simulink model "vehicle_body_revised"  (R2020b)
settings: Solver=VariableStepAuto  StartTime=0.0  StopTime=10.0  RelTol=1e-3
libraries: sdl_lib x17, nesl_utility x8, autolibdatasheetbattery x1, autolibmappedmotor x1
settings Model: Creator=True  LastModifiedBy=True

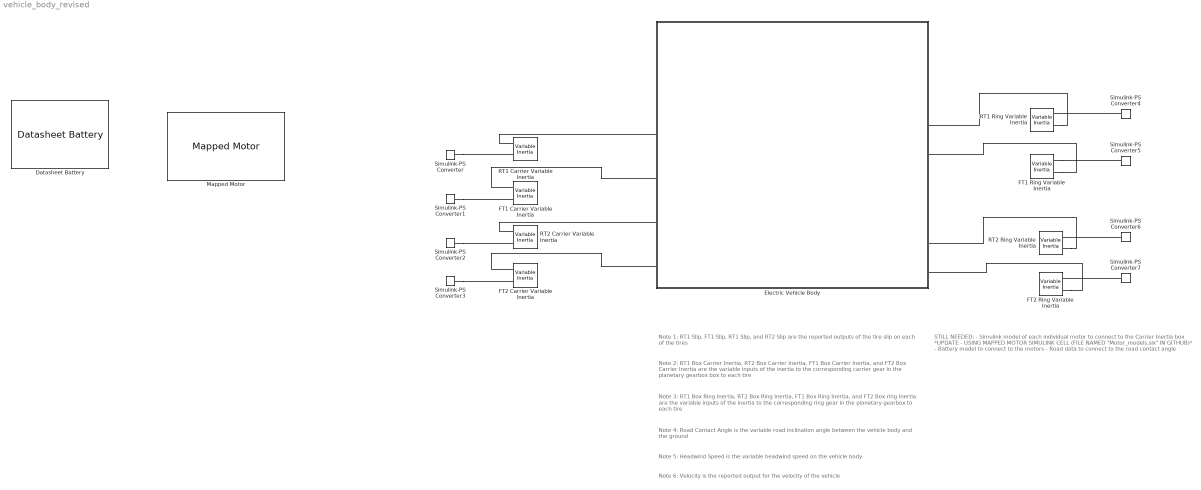
== system vehicle_body_revised ==
  note: STILL NEEDED:
      | - Simulink model of each individual motor to connect to the Carrier Inertia box *UPDATE - USING MAPPED MOTOR SIMULINK CELL (FILE NAMED "Motor_models.slx" IN GITHUB)*
      |
      | - Battery model to connect to the motors
      |
      | - Road data to connect to the road contact angle
  note: Note 6: Velocity is the reported output for the velocity of the vehicle
  note: Note 5: Headwind Speed is the variable headwind speed on the vehicle body
  note: Note 4: Road Contact Angle is the variable road inclination angle between the vehicle body and the ground
  note: Note 3: RT1 Box Ring Inertia, RT2 Box Ring Inertia, FT1 Box Ring Inertia, and FT2 Box ring Inertia are the variable inputs of the inertia to the corresponding ring gear in the planetary gearbox to each tire
  note: Note 2: RT1 Box Carrier Inertia, RT2 Box Carrier Inertia, FT1 Box Carrier Inertia, and FT2 Box Carrier Inertia are the variable inputs of the inertia to the corresponding carrier gear in the planetary gearbox box to each tire
  note: Note 1: RT1 Slip, FT1 Slip, RT1 Slip, and RT2 Slip are the reported outputs of the tire slip on each of the tires
  Datasheet Battery : autolibdatasheetbattery/Datasheet Battery  CapacityCtrl=Parameter  OutputVlt=Unfiltered  BattChargeMax=100  Em=[2.8 3.228 3.284 3.361 3.408 3.427 3.472 3.477 3.493 3.504 3.516 3.528 3.537 3.545 3.555 3.561 3.566 3.576 3.587 3.589 3.594 3.6 3.608 3.61 3.616 3.619 3.626 3.632 3.637 3.64 3.645 3.646 3.652 3.655 3.658 3.661 3.664 3.668 3.673 3.678 3.68 3.681 3.686 3.692 3.699 3.702 3.705 3.71 3.717 3.723 3.728 3.733 3.735 3.742 3.749 3.755 3.761 3.768 3.773 3.78 3.791 3.798 3.798 3.814 3.818 3.825 3.841 3.846 3.855 3.863 3.877 3.885 3.894 3.907 3.919 3.926 3.935 3.944 3.954 3.964 3.974 3.988 3.998 4.014 4.029 4.034 4.047 4.065 4.074 4.086 4.097 4.131 4.126 4.138 4.15 4.18 4.174 4.187 4.207 4.231 4.221]  CapLUTBp=[0 0.01 0.02 0.03 0.04 0.05 0.06 0.07 0.08 0.09 0.1 0.11 0.12 0.13 0.14 0.15 0.16 0.17 0.18 0.19 0.2 0.21 0.22 0.23 0.24 0.25 0.26 0.27 0.28 0.29 0.3 0.31 0.32 0.33 0.34 0.35 0.36 0.37 0.38 0.39 0.4 0.41 0.42 0.43 0.44 0.45 0.46 0.47 0.48 0.49 0.5 0.51 0.52 0.53 0.54 0.55 0.56 0.57 0.58 0.59 0.6 0.61 0.62 0.63 0.64 0.65 0.66 0.67 0.68 0.69 0.7 0.71 0.72 0.73 0.74 0.75 0.76 0.77 0.78 0.79 0.8 0.81 0.82 0.83 0.84 0.85 0.86 0.87 0.88 0.89 0.9 0.91 0.92 0.93 0.94 0.95 0.96 0.97 0.98 0.99 1]  RInt=[0.008846 0.009319 0.009027 0.00847 0.01032 0.01314;0.006389 0.006554 0.005553 0.005525 0.006043 0.007805;0.004364 0.004101 0.00406 0.003452 0.003846 0.004517;0.002031 0.002563 0.002532 0.00246 0.002716 0.003047;0.001443 0.001825 0.001795 0.001778 0.001924 0.002234;0.0005603 0.0007192 0.0006887 0.0007557 0.0007355 0.001014;0.001028 0.001338 0.001 0.001536 0.001546 0.002789]  BattTempBp=[243.1 253.1 263.1 273.1 283.1 298.1 313.1]  CapSOCBp=[0 0.2 0.4 0.6 0.8 1]  Ns=1  Np=1  BattCapInit=100  Tc=1/1000  Vinit=4.221  RefBlkName='autolibdatasheetbattery/Datasheet Battery'
      settings: SourceProductBaseCode=PW
  Electric Vehicle Body : Subsystem
  FT1 Carrier Variable Inertia : sdl_lib/Inertias & Loads/Variable Inertia  minimum_inertia=0.1 kg*m^2  L_specify=off  L_priority=High  L=0 m^2*kg/s  L_nominal_specify=off  L_nominal_unit=m^2*kg/s  L_nominal_value=1
      settings: SourceProductBaseCode=LD  InternalSimscapePortConfiguration="{\"Bottom\":[],\"Left\":[{\"id\":\"I\",\"label\":\"\",\"type\":\"input\"},{\"id\":\"A\",\"label\":\"\",\"type\":\"foundation.mechanical.rotational.rotational\"}],\"Right\":[],\"Top\":[]}"
  FT1 Ring Variable Inertia : sdl_lib/Inertias & Loads/Variable Inertia  minimum_inertia=0.1 kg*m^2  L_specify=off  L_priority=High  L=0 m^2*kg/s  L_nominal_specify=off  L_nominal_unit=m^2*kg/s  L_nominal_value=1
      settings: SourceProductBaseCode=LD  InternalSimscapePortConfiguration="{\"Bottom\":[],\"Left\":[{\"id\":\"I\",\"label\":\"\",\"type\":\"input\"},{\"id\":\"A\",\"label\":\"\",\"type\":\"foundation.mechanical.rotational.rotational\"}],\"Right\":[],\"Top\":[]}"
  FT2 Carrier Variable Inertia : sdl_lib/Inertias & Loads/Variable Inertia  minimum_inertia=0.1 kg*m^2  L_specify=off  L_priority=High  L=0 m^2*kg/s  L_nominal_specify=off  L_nominal_unit=m^2*kg/s  L_nominal_value=1
      settings: SourceProductBaseCode=LD  InternalSimscapePortConfiguration="{\"Bottom\":[],\"Left\":[{\"id\":\"I\",\"label\":\"\",\"type\":\"input\"},{\"id\":\"A\",\"label\":\"\",\"type\":\"foundation.mechanical.rotational.rotational\"}],\"Right\":[],\"Top\":[]}"
  FT2 Ring Variable Inertia : sdl_lib/Inertias & Loads/Variable Inertia  minimum_inertia=0.1 kg*m^2  L_specify=off  L_priority=High  L=0 m^2*kg/s  L_nominal_specify=off  L_nominal_unit=m^2*kg/s  L_nominal_value=1
      settings: SourceProductBaseCode=LD  InternalSimscapePortConfiguration="{\"Bottom\":[],\"Left\":[{\"id\":\"I\",\"label\":\"\",\"type\":\"input\"},{\"id\":\"A\",\"label\":\"\",\"type\":\"foundation.mechanical.rotational.rotational\"}],\"Right\":[],\"Top\":[]}"
  Mapped Motor : autolibmappedmotor/Mapped Motor  port_config=Torque  param_by=Tabulated torque-speed envelope  w_t=[ 0 375 750 800 ]  T_t=[0.09 0.08 0.07 0]  torque_max=.1  power_max=30  Tc=0.02  param_loss=Single efficiency measurement  eff=100  w_eff=375  T_eff=0.08  Piron=0  Pbase=0  w_eff_bp=[-8000 -4000 0 4000 8000]  T_eff_bp=[0 0.03 0.06 0.09]  Temp_eff_bp=[233.15 293.15 373.15]  losses_table=[1.49 1.67 2.21 3.10; 0.42 0.69 1.14 2.03; 0.06 0.24 0.78 1.68; 0.42 0.69 1.14 2.03; 1.49 1.67 2.21 3.10]  losses_table_3d=cat(3,[1.49 1.67 2.21 3.10; 0.42 0.69 1.14 2.03; 0.06 0.24 0.78 1.68; 0.42 0.69 1.14 2.03; 1.49 1.67 2.21 3.10],[1.49 1.67 2.21 3.10; 0.42 0.69 1.14 2.03; 0.06 0.24 0.78 1.68; 0.42 0.69 1.14 2.03; 1.49 1.67 2.21 3.10],[1.49 1.67 2.21 3.10; 0.42 0.69 1.14 2.03; 0.06 0.24 0.78 1.68; 0.42 0.69 1.14 2.03; 1.49 1.67 2.21 3.10])  efficiency_table=[95 95 95 95; 95 95 95 95; 95 95 95 95; 95 95 95 95; 95 95 95 95]  efficiency_table_3d=cat(3,[95 95 95 95; 95 95 95 95; 95 95 95 95; 95 95 95 95; 95 95 95 95],[95 95 95 95; 95 95 95 95; 95 95 95 95; 95 95 95 95; 95 95 95 95],[95 95 95 95; 95 95 95 95; 95 95 95 95; 95 95 95 95; 95 95 95 95])  J=5e-6  b=1e-5  omega_o=0  T_t_extended=[0 0.07 0.08 0.09 0.08 0.07 0]  w_t_extended=[-800 -750 -375 0 375 750 800]  KLossIron=0  KLossCopper=0  x_w_eff_vec=[-8000 -4000 0 4000 8000]  x_T_eff_vec=[-0.09 -0.06 -0.03 0 0.03 0.06 0.09]  x_tmp_eff_vec=[-0.09 -0.06 -0.03 0 0.03 0.06 0.09]  x_losses_mat=[3.1 2.21 1.67 1.49 1.67 2.21 3.1;2.03 1.14 0.69 0.42 0.69 1.14 2.03;1.68 0.78 0.24 0.06 0.24 0.78 1.68;2.03 1.14 0.69 0.42 0.69 1.14 2.03;3.1 2.21 1.67 1.49 1.67 2.21 3.1]  x_losses_mat_3d=[37.8947368421052 25.2631578947368 12.6315789473684 0 12 24 36;18.9473684210526 12.6315789473684 6.3157894736842 0 5.99999999999999 12 18;0 0 0 0 0 0 0;18 12 5.99999999999999 0 6.3157894736842 12.6315789473684 18.9473684210526;36 24 12 0 12.6315789473684 25.2631578947368 37.8947368421052]  CalLossMapData={}  CalLossWithTempMapData={}  aMode=1  RefBlkName='autolibmappedmotor/Mapped Motor'
      settings: SourceProductBaseCode=PW,MT,UV,VE,VP
  RT1 Carrier Variable Inertia : sdl_lib/Inertias & Loads/Variable Inertia  minimum_inertia=0.1 kg*m^2  L_specify=off  L_priority=High  L=0 m^2*kg/s  L_nominal_specify=off  L_nominal_unit=m^2*kg/s  L_nominal_value=1
      settings: SourceProductBaseCode=LD  InternalSimscapePortConfiguration="{\"Bottom\":[],\"Left\":[{\"id\":\"I\",\"label\":\"\",\"type\":\"input\"},{\"id\":\"A\",\"label\":\"\",\"type\":\"foundation.mechanical.rotational.rotational\"}],\"Right\":[],\"Top\":[]}"
  RT1 Ring Variable Inertia : sdl_lib/Inertias & Loads/Variable Inertia  minimum_inertia=0.1 kg*m^2  L_specify=off  L_priority=High  L=0 m^2*kg/s  L_nominal_specify=off  L_nominal_unit=m^2*kg/s  L_nominal_value=1
      settings: SourceProductBaseCode=LD  InternalSimscapePortConfiguration="{\"Bottom\":[],\"Left\":[{\"id\":\"I\",\"label\":\"\",\"type\":\"input\"},{\"id\":\"A\",\"label\":\"\",\"type\":\"foundation.mechanical.rotational.rotational\"}],\"Right\":[],\"Top\":[]}"
  RT2 Carrier Variable Inertia : sdl_lib/Inertias & Loads/Variable Inertia  minimum_inertia=0.1 kg*m^2  L_specify=off  L_priority=High  L=0 m^2*kg/s  L_nominal_specify=off  L_nominal_unit=m^2*kg/s  L_nominal_value=1
      settings: SourceProductBaseCode=LD  InternalSimscapePortConfiguration="{\"Bottom\":[],\"Left\":[{\"id\":\"I\",\"label\":\"\",\"type\":\"input\"},{\"id\":\"A\",\"label\":\"\",\"type\":\"foundation.mechanical.rotational.rotational\"}],\"Right\":[],\"Top\":[]}"
  RT2 Ring Variable Inertia : sdl_lib/Inertias & Loads/Variable Inertia  minimum_inertia=0.1 kg*m^2  L_specify=off  L_priority=High  L=0 m^2*kg/s  L_nominal_specify=off  L_nominal_unit=m^2*kg/s  L_nominal_value=1
      settings: SourceProductBaseCode=LD  InternalSimscapePortConfiguration="{\"Bottom\":[],\"Left\":[{\"id\":\"I\",\"label\":\"\",\"type\":\"input\"},{\"id\":\"A\",\"label\":\"\",\"type\":\"foundation.mechanical.rotational.rotational\"}],\"Right\":[],\"Top\":[]}"
  Simulink-PS Converter{,1..7} (8 alike) : nesl_utility/Simulink-PS Converter  PhysicalDomain=network_engine_domain  SubClassName=ps_input  LeftPortType=input  RightPortType=output  PseudoPeriodic=off  Frequencies=[]  NoiseDistribution=none  NoiseParameters=[]  Unit=1  AffineConversion=off  FilteringAndDerivatives=provide  SimscapeFilterOrder=1  InputFilterTimeConstant=0.001  UdotUserProvided=0
  connections:
  RT1 Carrier Variable Inertia/LConn2 -- Electric Vehicle Body/LConn3
  FT1 Carrier Variable Inertia/LConn2 -- Electric Vehicle Body/LConn4
  RT2 Carrier Variable Inertia/LConn2 -- Electric Vehicle Body/LConn5
  FT2 Carrier Variable Inertia/LConn2 -- Electric Vehicle Body/LConn6
  RT1 Ring Variable Inertia/LConn2 -- Electric Vehicle Body/RConn4
  FT1 Ring Variable Inertia/LConn2 -- Electric Vehicle Body/RConn5
  RT2 Ring Variable Inertia/LConn2 -- Electric Vehicle Body/RConn8
  FT2 Ring Variable Inertia/LConn2 -- Electric Vehicle Body/RConn9
  Simulink-PS Converter/RConn1 -- RT1 Carrier Variable Inertia/LConn1
  Simulink-PS Converter1/RConn1 -- FT1 Carrier Variable Inertia/LConn1
  Simulink-PS Converter2/RConn1 -- RT2 Carrier Variable Inertia/LConn1
  Simulink-PS Converter3/RConn1 -- FT2 Carrier Variable Inertia/LConn1
  Simulink-PS Converter4/RConn1 -- RT1 Ring Variable Inertia/LConn1
  FT1 Ring Variable Inertia/LConn1 -- Simulink-PS Converter5/RConn1
  Simulink-PS Converter6/RConn1 -- RT2 Ring Variable Inertia/LConn1
  Simulink-PS Converter7/RConn1 -- FT2 Ring Variable Inertia/LConn1

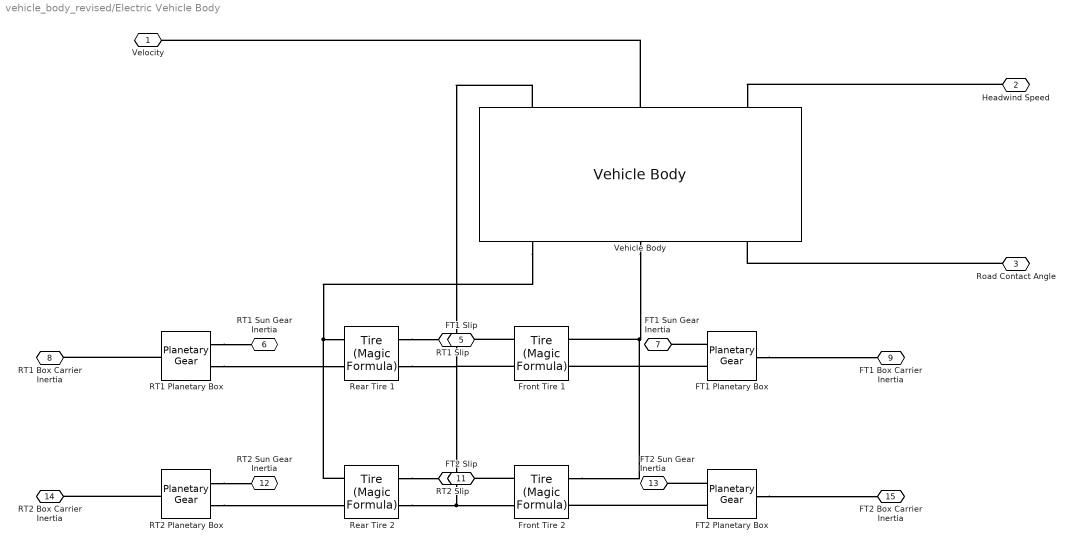
== system vehicle_body_revised/Electric Vehicle Body ==
  FT1 Planetary Box : sdl_lib/Gears/Planetary Gear  rs_ratio=2  friction_model=sdl.enum.gear_friction.none  mu_visc=[0, 0] N*m/(rad/s)  efficiency=[.96, .98]  temperature_TLU=[280, 300, 320] K  efficiency_sp_TLU=[.95, .9, .85]  efficiency_rp_TLU=[.95, .9, .85]  pwr_thr=[.001, .001] W  thermal_mass=50 J/K  T_init=300 K  model_inertia=simscape.enum.onoff.off  planet_inertia=0.001 kg*m^2
      settings: SourceProductBaseCode=LD
  FT2 Planetary Box : sdl_lib/Gears/Planetary Gear  rs_ratio=2  friction_model=sdl.enum.gear_friction.none  mu_visc=[0, 0] N*m/(rad/s)  efficiency=[.96, .98]  temperature_TLU=[280, 300, 320] K  efficiency_sp_TLU=[.95, .9, .85]  efficiency_rp_TLU=[.95, .9, .85]  pwr_thr=[.001, .001] W  thermal_mass=50 J/K  T_init=300 K  model_inertia=simscape.enum.onoff.off  planet_inertia=0.001 kg*m^2
      settings: SourceProductBaseCode=LD
  Front Tire 1 : sdl_lib/Tires & Vehicles/Tire (Magic Formula)  parameterization=sdl.enum.magic_tire_model.peak  F_z1=3000 N  F_x1=3500 N  kappa1=10  B_m=10  C_m=1.9  D_m=1  E_m=0.97  fz0=4000 N  p_Cx=1.685  p_Dx=[1.21, -.037]  p_Ex=[.344, .095, -.02, 0]  p_Kx=[21.51, -.163, .245]  p_Hx=[-.002, .002]  p_Vx=[0, 0]  v_tr_thr=0.1 m/s  r_e=0.3 m  model_compliance=0  stiffness=1e6 N/m  damping=1000 N/(m/s)  model_inertia=0  inertia=1 kg*m^2  initial_velocity=0 rad/s  model_resistance=0  resistance_model=1  coeff=0.015  p_tire=250e3 Pa  alpha=-0.003  beta=0.97  coeff_a=84e-4  coeff_b=6.2e-4 s/m  coeff_c=1.6e-4 s^2/m^2  v_thr=0.001 m/s
  Front Tire 2 : sdl_lib/Tires & Vehicles/Tire (Magic Formula)  parameterization=sdl.enum.magic_tire_model.peak  F_z1=3000 N  F_x1=3500 N  kappa1=10  B_m=10  C_m=1.9  D_m=1  E_m=0.97  fz0=4000 N  p_Cx=1.685  p_Dx=[1.21, -.037]  p_Ex=[.344, .095, -.02, 0]  p_Kx=[21.51, -.163, .245]  p_Hx=[-.002, .002]  p_Vx=[0, 0]  v_tr_thr=0.1 m/s  r_e=0.3 m  model_compliance=0  stiffness=1e6 N/m  damping=1000 N/(m/s)  model_inertia=0  inertia=1 kg*m^2  initial_velocity=0 rad/s  model_resistance=0  resistance_model=1  coeff=0.015  p_tire=250e3 Pa  alpha=-0.003  beta=0.97  coeff_a=84e-4  coeff_b=6.2e-4 s/m  coeff_c=1.6e-4 s^2/m^2  v_thr=0.001 m/s
  RT1 Planetary Box : sdl_lib/Gears/Planetary Gear  rs_ratio=2  friction_model=sdl.enum.gear_friction.none  mu_visc=[0, 0] N*m/(rad/s)  efficiency=[.96, .98]  temperature_TLU=[280, 300, 320] K  efficiency_sp_TLU=[.95, .9, .85]  efficiency_rp_TLU=[.95, .9, .85]  pwr_thr=[.001, .001] W  thermal_mass=50 J/K  T_init=300 K  model_inertia=simscape.enum.onoff.off  planet_inertia=0.001 kg*m^2
      settings: SourceProductBaseCode=LD
  RT2 Planetary Box : sdl_lib/Gears/Planetary Gear  rs_ratio=2  friction_model=sdl.enum.gear_friction.none  mu_visc=[0, 0] N*m/(rad/s)  efficiency=[.96, .98]  temperature_TLU=[280, 300, 320] K  efficiency_sp_TLU=[.95, .9, .85]  efficiency_rp_TLU=[.95, .9, .85]  pwr_thr=[.001, .001] W  thermal_mass=50 J/K  T_init=300 K  model_inertia=simscape.enum.onoff.off  planet_inertia=0.001 kg*m^2
      settings: SourceProductBaseCode=LD
  Rear Tire 1 : sdl_lib/Tires & Vehicles/Tire (Magic Formula)  parameterization=sdl.enum.magic_tire_model.peak  F_z1=3000 N  F_x1=3500 N  kappa1=10  B_m=10  C_m=1.9  D_m=1  E_m=0.97  fz0=4000 N  p_Cx=1.685  p_Dx=[1.21, -.037]  p_Ex=[.344, .095, -.02, 0]  p_Kx=[21.51, -.163, .245]  p_Hx=[-.002, .002]  p_Vx=[0, 0]  v_tr_thr=0.1 m/s  r_e=0.3 m  model_compliance=0  stiffness=1e6 N/m  damping=1000 N/(m/s)  model_inertia=0  inertia=1 kg*m^2  initial_velocity=0 rad/s  model_resistance=0  resistance_model=1  coeff=0.015  p_tire=250e3 Pa  alpha=-0.003  beta=0.97  coeff_a=84e-4  coeff_b=6.2e-4 s/m  coeff_c=1.6e-4 s^2/m^2  v_thr=0.001 m/s
  Rear Tire 2 : sdl_lib/Tires & Vehicles/Tire (Magic Formula)  parameterization=sdl.enum.magic_tire_model.peak  F_z1=3000 N  F_x1=3500 N  kappa1=10  B_m=10  C_m=1.9  D_m=1  E_m=0.97  fz0=4000 N  p_Cx=1.685  p_Dx=[1.21, -.037]  p_Ex=[.344, .095, -.02, 0]  p_Kx=[21.51, -.163, .245]  p_Hx=[-.002, .002]  p_Vx=[0, 0]  v_tr_thr=0.1 m/s  r_e=0.3 m  model_compliance=0  stiffness=1e6 N/m  damping=1000 N/(m/s)  model_inertia=0  inertia=1 kg*m^2  initial_velocity=0 rad/s  model_resistance=0  resistance_model=1  coeff=0.015  p_tire=250e3 Pa  alpha=-0.003  beta=0.97  coeff_a=84e-4  coeff_b=6.2e-4 s/m  coeff_c=1.6e-4 s^2/m^2  v_thr=0.001 m/s
  Vehicle Body : sdl_lib/Tires & Vehicles/Vehicle Body  mass=1200 kg  n_w=2  x_f=1.4 m  x_r=1.6 m  y_c=0.5 m  mass_var=simscape.enum.onoff.off  model_pitch=simscape.enum.onoff.off  inertia=4000 kg*m^2  suspension_model=sdl.enum.linearTLU.linear  k_f=1e4 N/m  b_f=1e4 N/(m/s)  k_r=1e4 N/m  b_r=1e4 N/(m/s)  k_f_TLU=[-2000, -1000, 0, 1000, 2000] N  x_f_TLU=[-.4, -.2, 0, .2, .4] m  b_f_TLU=[-200, -100, 0, 100, 200] N  v_f_TLU=[-4, -2, 0, 2, 4] m/s  k_r_TLU=[-2000, -1000, 0, 1000, 2000] N  x_r_TLU=[-.4, -.2, 0, .2, .4] m  b_r_TLU=[-200, -100, 0, 100, 200] N  v_r_TLU=[-4, -2, 0, 2, 4] m/s  interp_method=simscape.enum.interpolation.linear  extrap_method=simscape.enum.extrapolation.linear  model_hardstop=simscape.enum.onoff.off  upper_bound_f=.25 m  lower_bound_f=-.25 m  stop_k_f=1e6 N/m  stop_b_f=150 N/(m/s)  upper_bound_r=.25 m  lower_bound_r=-.25 m  stop_k_r=1e6 N/m  stop_b_r=150 N/(m/s)  initial_pitch=0 rad  initial_pitch_rate=0 rad/s  g=9.81 m/s^2  liftoff_warning=simscape.enum.onoff.off  area=3 m^2  Cd=0.4  rho=1.18 kg/m^3  v_specify=off  v_priority=High  v=0 m/s  v_nominal_specify=off  v_nominal_unit=m/s  v_nominal_value=1
  Velocity : PMIOPort  Side=Left
  Headwind Speed : PMIOPort  Port=2  Side=Left
  Road Contact Angle : PMIOPort  Port=3  Side=Right
  RT1 Slip : PMIOPort  Port=4  Side=Right
  FT1 Slip : PMIOPort  Port=5  Side=Right
  RT1 Sun Gear Inertia : PMIOPort  Port=6  Side=Right
  FT1 Sun Gear Inertia : PMIOPort  Port=7  Side=Right
  RT1 Box Carrier Inertia : PMIOPort  Port=8  Side=Left
  FT1 Box Carrier Inertia : PMIOPort  Port=9  Side=Left
  RT2 Slip : PMIOPort  Port=10  Side=Right
  FT2 Slip : PMIOPort  Port=11  Side=Right
  RT2 Sun Gear Inertia : PMIOPort  Port=12  Side=Right
  FT2 Sun Gear Inertia : PMIOPort  Port=13  Side=Right
  RT2 Box Carrier Inertia : PMIOPort  Port=14  Side=Left
  FT2 Box Carrier Inertia : PMIOPort  Port=15  Side=Left
  connections:
  Front Tire 2/LConn1 -- Front Tire 1/LConn1 -- Vehicle Body/RConn2
  Rear Tire 2/LConn1 -- Rear Tire 1/LConn1 -- Vehicle Body/RConn1
  Road Contact Angle/RConn1 -- Vehicle Body/RConn3
  FT2 Planetary Box/RConn2 -- Front Tire 2/LConn2
  Rear Tire 2/RConn2 -- Front Tire 2/RConn2 -- Rear Tire 1/RConn2 -- Front Tire 1/RConn2 -- Vehicle Body/LConn1
  FT1 Planetary Box/RConn2 -- Front Tire 1/LConn2
  RT2 Planetary Box/LConn1 -- RT2 Box Carrier Inertia/RConn1
  RT2 Planetary Box/RConn1 -- Rear Tire 2/LConn2
  RT1 Planetary Box/RConn1 -- Rear Tire 1/LConn2
  Rear Tire 1/RConn1 -- RT1 Slip/RConn1
  Front Tire 1/RConn1 -- FT1 Slip/RConn1
  FT1 Planetary Box/LConn1 -- FT1 Box Carrier Inertia/RConn1
  RT1 Planetary Box/RConn2 -- RT1 Sun Gear Inertia/RConn1
  RT1 Planetary Box/LConn1 -- RT1 Box Carrier Inertia/RConn1
  Headwind Speed/RConn1 -- Vehicle Body/LConn3
  FT1 Planetary Box/RConn1 -- FT1 Sun Gear Inertia/RConn1
  RT2 Planetary Box/RConn2 -- RT2 Sun Gear Inertia/RConn1
  Front Tire 2/RConn1 -- FT2 Slip/RConn1
  Vehicle Body/LConn2 -- Velocity/RConn1
  FT2 Planetary Box/RConn1 -- FT2 Sun Gear Inertia/RConn1
  Rear Tire 2/RConn1 -- RT2 Slip/RConn1
  FT2 Planetary Box/LConn1 -- FT2 Box Carrier Inertia/RConn1
